simulink model "ex3p3"  (R2016b)
settings: Solver=VariableStepAuto  StartTime=0.0  StopTime=1.5  RelTol=1e-3
InitFcn:
  | alpha=0;
libraries: powerlib x10, powerlib_meascontrol x4, simulink x4
settings Model: Creator=user  LastModifiedBy=user

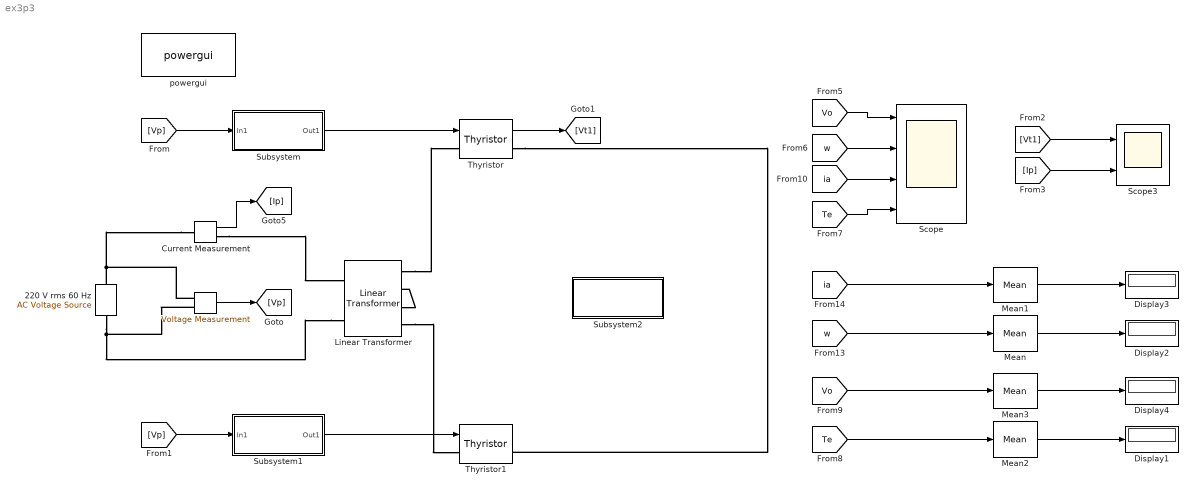
== system ex3p3 ==
  " " : powerlib/Measurements/Voltage Measurement  PhasorSimulation=off  OutputType=Complex  PSBequivalent=0
  220 V rms 60 Hz : powerlib/Electrical Sources/AC Voltage Source  Amplitude=220*sqrt(2)  Phase=0  Frequency=60  SampleTime=0  Measurements=None  BusType=swing  Pref=10e3  Qref=0  Qmin=-inf  Qmax=+inf
  Current Measurement : powerlib/Measurements/Current Measurement  PhasorSimulation=off  OutputType=Complex  PSBequivalent=0
  Display{1..4} (4 alike) : Display
  Linear Transformer : powerlib/Elements/Linear Transformer  UNITS=pu  NominalPower=[ 100e3 60 ]  winding1="[220  0.002  0.08 ]"  winding2="[266.5  0.002  0.08 ]"  ThreeWindings=on  winding3=[266.5 0.002 0.08 ]  RmLm=[ 500 500 ]  Measurements=None  DataType=off
  Mean{,1..3} (4 alike) : powerlib_meascontrol/Measurements/Mean  Freq=60  Vinit=0  Ts=0
  Scope : Scope  NumInputPorts=4
  Scope3 : Scope  NumInputPorts=2
  Subsystem : Subsystem
  Subsystem1 : Subsystem
  Subsystem2 : Subsystem
  Thyristor : powerlib/Power Electronics/Thyristor  Ron=0.001  Lon=0  Vf=0.8  IC=0  Rs=500  Cs=250e-9  Measurements=on
  Thyristor1 : powerlib/Power Electronics/Thyristor  Ron=0.001  Lon=0  Vf=0.8  IC=0  Rs=500  Cs=250e-9  Measurements=on
  powergui : powerlib/powergui  Priority=1  SimulationMode=Continuous  SolverType=Tustin/Backward Euler (TBE)  SampleTime=50e-6  frequency=60  SPID=off  DisableSnubberDevices=off  DisableRonSwitches=off  DisableVfSwitches=off  SwTol=0  DisplayEquations=off  Interpol=off  ExternalGateDelay=off  methode=off  Ts=10  FunctionMessages=off  echomessages=off  HookPort=off  EnableUseOfTLC=off  x0status=blocks  frequencyindice=60  Pbase=100e6  ErrMax=1e-4  Iterations=50  UnitsV=kV  UnitsW=MW  buscounter=0  RestoreLinks=warning  ResistiveCurrentMeasurement=off  Frange=[0:2:500]  Ylog=off  Xlog=on  ShowGrid=off  save=off  variable=ZData  structure=0  ZoomFFT=off  StartTime=0.0  cycles=1  DisplayStyle=1  fundamental=60  FreqAxis=off  MaxFrequency=1000  frequencyindicesteady=1  RmsSteady=1  display=off
  wires:
  Subsystem/1(Out1) -> Thyristor/1
  Subsystem1/1(Out1) -> Thyristor1/1
  " "/1 -> [Vp]
  [Vp] -> Subsystem1/1(In1)
  [Vp] -> Subsystem/1(In1)
  Thyristor/1 -> [Vt1]
  Current Measurement/1 -> [Ip]
  [Vt1] -> Scope3/1
  [Ip] -> Scope3/2
  [Vo] -> Scope/1
  [w] -> Scope/2
  [ia] -> Scope/3
  Mean1/1 -> Display3/1
  Mean/1 -> Display2/1
  [ia] -> Mean1/1
  [w] -> Mean/1
  [Te] -> Scope/4
  Mean3/1 -> Display4/1
  Mean2/1 -> Display1/1
  [Vo] -> Mean3/1
  [Te] -> Mean2/1
  connections:
  Current Measurement/LConn1 -- " "/LConn1 -- 220 V rms 60 Hz/RConn1
  Linear Transformer/LConn2 -- " "/LConn2 -- 220 V rms 60 Hz/LConn1
  Linear Transformer/RConn3 -- Linear Transformer/RConn2
  Linear Transformer/RConn1 -- Thyristor/LConn1
  Thyristor/RConn1 -- Thyristor1/RConn1
  Linear Transformer/RConn4 -- Thyristor1/LConn1
  Current Measurement/RConn1 -- Linear Transformer/LConn1

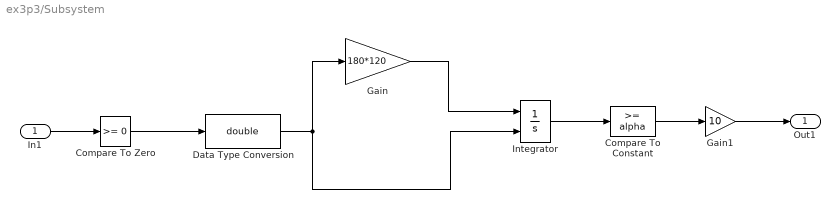
== system ex3p3/Subsystem ==
  In1 : Inport
  Compare To Constant : simulink/Logic and Bit Operations/Compare To Constant  relop=>=  const=alpha  OutDataTypeStr=boolean
  Compare To Zero : simulink/Logic and Bit Operations/Compare To Zero  relop=>=  OutDataTypeStr=boolean
  Data Type Conversion : DataTypeConversion  OutDataTypeStr=double
  Gain : Gain  Gain=180*120
  Gain1 : Gain  Gain=10
  Integrator : Integrator  ExternalReset=falling
  Out1 : Outport
  wires:
  In1/1 -> Compare To Zero/1
  Compare To Zero/1 -> Data Type Conversion/1
  Gain/1 -> Integrator/1
  Data Type Conversion/1 -> Gain/1, Integrator/2
  Integrator/1 -> Compare To Constant/1
  Compare To Constant/1 -> Gain1/1
  Gain1/1 -> Out1/1

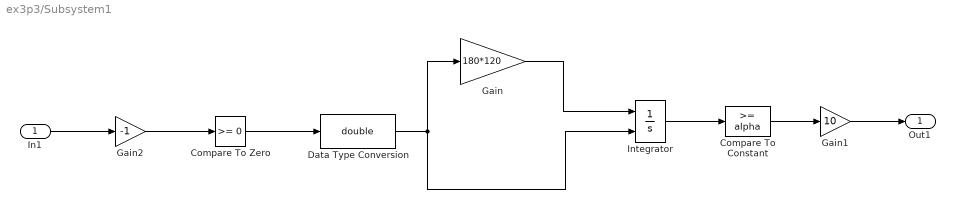
== system ex3p3/Subsystem1 ==
  In1 : Inport
  Compare To Constant : simulink/Logic and Bit Operations/Compare To Constant  relop=>=  const=alpha  OutDataTypeStr=boolean
  Compare To Zero : simulink/Logic and Bit Operations/Compare To Zero  relop=>=  OutDataTypeStr=boolean
  Data Type Conversion : DataTypeConversion  OutDataTypeStr=double
  Gain : Gain  Gain=180*120
  Gain1 : Gain  Gain=10
  Gain2 : Gain  Gain=-1
  Integrator : Integrator  ExternalReset=falling
  Out1 : Outport
  wires:
  Compare To Zero/1 -> Data Type Conversion/1
  Gain/1 -> Integrator/1
  Data Type Conversion/1 -> Gain/1, Integrator/2
  Integrator/1 -> Compare To Constant/1
  Compare To Constant/1 -> Gain1/1
  Gain1/1 -> Out1/1
  In1/1 -> Gain2/1
  Gain2/1 -> Compare To Zero/1

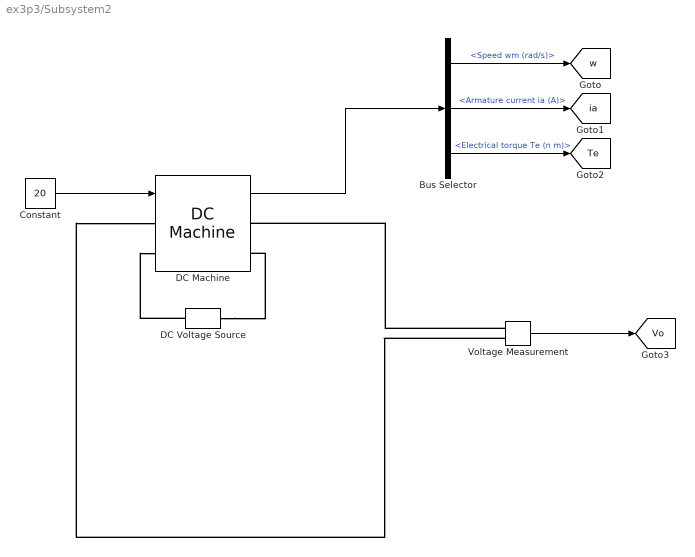
== system ex3p3/Subsystem2 ==
  Bus Selector : BusSelector  OutputSignals=Speed wm (rad/s),Armature current ia (A),Electrical torque Te (n m)
  Constant : Constant  Value=20
  DC Machine : powerlib/Machines/DC Machine  PresetModel=01: 5HP 240V 1750RPM Field:300V  MechanicalLoad=Torque TL  FieldType=Wound  ShowDetailedParameters=on  MeasurementBus=off  RLa=[2.581 0.028]  RLf=[281.3 156]  Laf=0.9483  MachineConstant=Torque constant (N.m/A)  Ke=1.8  Kt=1.8  J=0.02215  Bm=0.002953  Tf=0.5161  w0=1  Ifinit=1  TsPowergui=0  TsBlock=-1
  DC Voltage Source : powerlib/Electrical Sources/DC Voltage Source  Amplitude=300  Measurements=None
  Voltage Measurement : powerlib/Measurements/Voltage Measurement  PhasorSimulation=off  OutputType=Complex  PSBequivalent=0
  tag scope: Te=global, Vo=global, ia=global, w=global
  wires:
  Constant/1 -> DC Machine/1
  DC Machine/1 -> Bus Selector/1
  Bus Selector/1 -> [w]  "<Speed wm (rad/s)>"
  Bus Selector/3 -> [Te]  "<Electrical torque Te (n m)>"
  Bus Selector/2 -> [ia]  "<Armature current ia (A)>"
  Voltage Measurement/1 -> [Vo]
  connections:
  DC Voltage Source/RConn1 -- DC Machine/LConn2
  DC Voltage Source/LConn1 -- DC Machine/RConn2
  Voltage Measurement/LConn2 -- DC Machine/RConn1
  Voltage Measurement/LConn1 -- DC Machine/LConn1
